simulink model "finalpidsrm"  (R2023a)
settings: Solver=VariableStepAuto  StartTime=0.0  StopTime=10  RelTol=1e-3
undefined symbols (not defined in the file): DiscIntNeverNeededParam
libraries: spsDiodeLib x6, spsIGBTLib x6, spsDCVoltageSourceLib x1, slpidlib x1, spsSwitchedReluctanceMotorLib x1, sps_lib x1
settings Model: Creator=hp  LastModifiedBy=SAGNEEK SENGUPTA
settings SolverCC: ZeroCrossAlgorithm=Adaptive
settings DebuggingCC: IgnoredZcDiagnostic=none

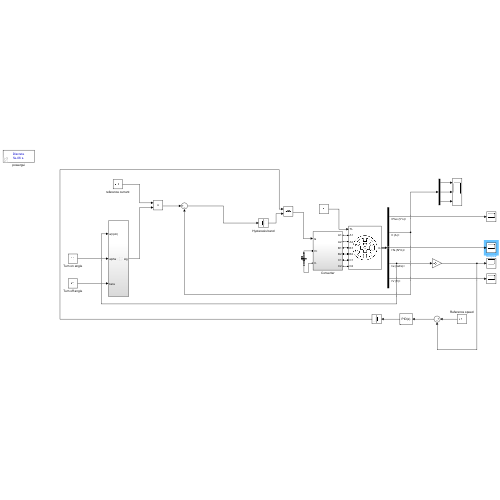
[thumbnail: Simulink's stored preview of the top-level diagram]
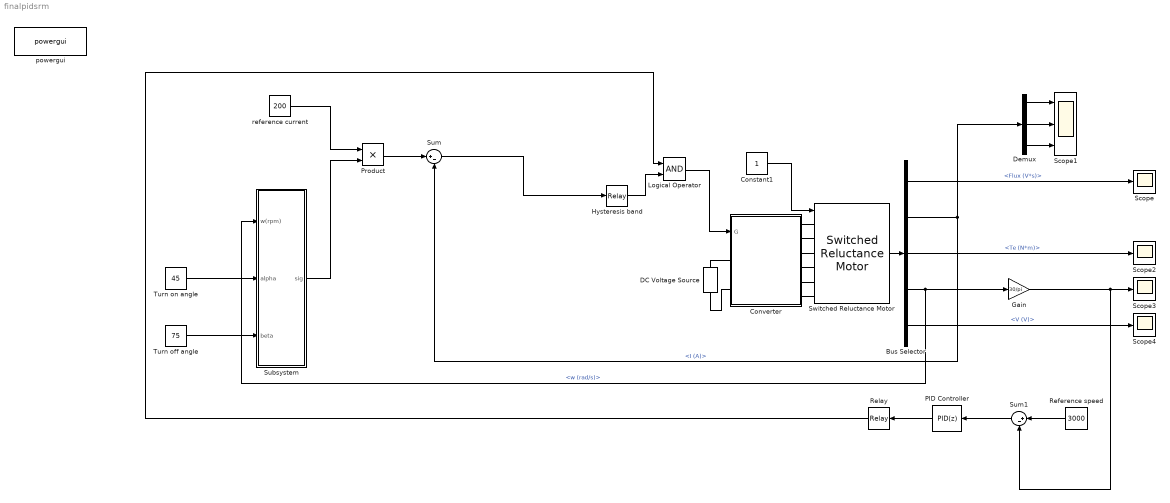
== system finalpidsrm ==
  Bus Selector : BusSelector  OutputSignals=Flux (V*s),I (A),Te (N*m),w (rad/s),V (V)
  Constant1 : Constant
  Converter : Subsystem
  DC Voltage Source : spsDCVoltageSourceLib/DC Voltage Source  Amplitude=240  Measurements=Voltage
  Demux : Demux  Outputs=3
  Gain : Gain  Gain=30/pi
  Hysteresis band : Relay  OnSwitchValue=10  OffSwitchValue=-10  ZeroCross=off
  Logical Operator : Logic  AllPortsSameDT=off  OutDataTypeStr=boolean
  PID Controller : slpidlib/PID Controller  Controller=PID  Form=Parallel  TimeDomain=Discrete-time  UseExternalTs=off  SampleTime=-1  IntegratorMethod=Forward Euler  FilterMethod=Forward Euler  ControllerParametersSource=internal  P=20  I=0.1  UseKiTs=off  D=0.05  N=100  UseFilter=on  TunerSelectOption=Transfer Function Based (PID Tuner App)  InitialConditionSource=internal  InitialConditionForIntegrator=0  InitialConditionForFilter=0  DifferentiatorICPrevScaledInput=0  ExternalReset=none  TrackingMode=off  Kt=1  LimitOutput=off  SatLimitsSource=internal  UpperSaturationLimit=inf  LowerSaturationLimit=-inf  LinearizeAsGain=on  AntiWindupMode=none  Kb=1  LimitIntegrator=off  UpperIntegratorSaturationLimit=inf  LowerIntegratorSaturationLimit=-inf  POutMin=[]  POutMax=[]  IOutMin=[]  IOutMax=[]  DOutMin=[]  DOutMax=[]  NOutMin=[]  NOutMax=[]  SumOutMin=[]  SumOutMax=[]  SaturationOutMin=[]  SaturationOutMax=[]  PParamMin=[]  PParamMax=[]  IParamMin=[]  IParamMax=[]  DParamMin=[]  DParamMax=[]  NParamMin=[]  NParamMax=[]  KbParamMin=[]  KbParamMax=[]  KtParamMin=[]  KtParamMax=[]  KbOutMin=[]  KbOutMax=[]  KtOutMin=[]  KtOutMax=[]  IntegratorOutMin=[]  IntegratorOutMax=[]  FilterOutMin=[]  FilterOutMax=[]  SumI1OutMin=[]  SumI1OutMax=[]  SumI2OutMin=[]  SumI2OutMax=[]  SumI3OutMin=[]  SumI3OutMax=[]  SumI4OutMin=[]  SumI4OutMax=[]  SumDOutMin=[]  SumDOutMax=[]  DifferentiatorOutMin=[]  DifferentiatorOutMax=[]  FilterDiffOutCoefMin=[]  FilterDiffOutCoefMax=[]  ReciprocalOutMin=[]  ReciprocalOutMax=[]  SumDenOutMin=[]  SumDenOutMax=[]  SumNumOutMin=[]  SumNumOutMax=[]  DivideOutMin=[]  DivideOutMax=[]  UdiffTsProdOutMin=[]  UdiffTsProdOutMax=[]  NTsProdOutMin=[]  NTsProdOutMax=[]  UintegralTsProdOutMin=[]  UintegralTsProdOutMax=[]  UngainTsProdOutMin=[]  UngainTsProdOutMax=[]  ClampingZeroOutDataTypeStr=Inherit: Inherit via back propagation  ClampingZeroOutMin=[]  ClampingZeroOutMax=[]  FilterDenConstantOutDataTypeStr=Inherit: Inherit via back propagation  FilterDenConstantOutMin=[]  FilterDenConstantOutMax=[]  PCopyOutDataTypeStr=Inherit: Inherit via back propagation  PCopyOutMin=[]  PCopyOutMax=[]  NCopyOutDataTypeStr=Inherit: Inherit via back propagation  NCopyOutMin=[]  NCopyOutMax=[]  IntegratorContinuousStateAttributes=''  IntegratorStateMustResolveToSignalObject=off  IntegratorRTWStateStorageClass=Auto  FilterContinuousStateAttributes=''  FilterStateMustResolveToSignalObject=off  FilterRTWStateStorageClass=Auto  ParallelPVariant=InternalParameters  IdealPVariant=Disabled  IVariant=InternalParameters  DVariant=InternalParameters  IntegratorVariant=Discrete  SatVariant=Disabled  AWVariant=Passthrough  PCopyVariant=Disabled  TRVariant=Disabled  FdbkBlocksVariant=Forward  IdealPFdbkVariant=Disabled  SatFdbkVariant=Disabled  DerivativeFilterVariant=ForwardEulerFilter  NVariant=InternalParameters  NCopyVariant=Disabled  FilterICVariant=InternalICsFilter  IntegratorICVariant=InternalICs  ExternalResetVariant=Disabled  TRSumVariant=Passthrough  SumFdbkVariant=Disabled  SumVariant=Sum_PID  TsampFilterVariant=InternalTs  TsampNgainVariant=Passthrough  TsampIntegralVariant=Disabled_SignalSpec  ExternalSaturationOutDataTypeStr=Inherit: Same as second input
  Product : Product
  Reference speed : Constant  Value=3000
  Relay : Relay
  Scope{,2..4} (4 alike) : Scope
  Scope1 : Scope  NumInputPorts=3
  Subsystem : Subsystem
  Sum : Sum  Inputs=|+-
  Sum1 : Sum  Inputs=|+-
  Switched Reluctance Motor : spsSwitchedReluctanceMotorLib/Switched Reluctance Motor  MachineType=6/4  StatorResistance=0.08  Inertia=0.0082  Friction=0.05  InitialSpeed=[0 0]  TsPowergui=0  TsBlock=-1  MachineModel=Generic model  Lq=0.67e-3  Ld=23.6e-3  Lsat=0.15e-3  MaximumCurrent=90  MaximumFluxLinkage=0.486  Source=MAT-file  MagnetisationCharacteristic='srm64_60kw.mat'  RotorAngleVector=[0 10 20 30 40 45]  StatorCurrentVector=[0:25:450]  PlotCurves=off
      settings: LibrarySourceBlock=|
      | sps_lib/Electrical Machines/Switched Reluctance
      | Motor
  Turn off angle : Constant  Value=75
  Turn on angle : Constant  Value=45
  powergui : sps_lib/powergui  Priority=1  SimulationMode=Discrete  SampleTime=5e-06  frequency=60  Iterations=50  frequencyindice=0  Pbase=100e6  ErrMax=1e-4  UnitsV=kV  UnitsW=MW  buscounter=0  FunctionMessages=off  echomessages=off  EnableUseOfTLC=off  CurrentSourceSwitches=off  DisableSnubberDevices=off  DisableRonSwitches=off  DisableVfSwitches=off  DisplayEquations=off  AutomaticDiscreteSolvers=off  SolverType=Tustin/Backward Euler (TBE)  Interpol=off  ExternalGateDelay=off  methode=off  Ts=100  x0status=blocks  SPID=on  SwTol=0  HookPort=off  NonlinearTolerance=1e-4  nMaxIteration=100  ContinueOnMaxIteration=off  RestoreLinks=warning  ResistiveCurrentMeasurement=off  Frange=[0:2:500]  Ylog=off  Xlog=on  ShowGrid=off  save=off  variable=ZData  structure=0  ZoomFFT=off  StartTime=0.0  cycles=1  DisplayStyle=1  fundamental=60  FreqAxis=off  MaxFrequency=1000  frequencyindicesteady=1  RmsSteady=1  display=off
  reference current : Constant  Value=200
  wires:
  Bus Selector/4 -> Subsystem/1(w(rpm)), Gain/1  "<w (rad/s)>"
  Gain/1 -> Scope3/1, Sum1/2
  Switched Reluctance Motor/1 -> Bus Selector/1
  Constant1/1 -> Switched Reluctance Motor/1
  Bus Selector/1 -> Scope/1  "<Flux (V*s)>"
  Bus Selector/2 -> Sum/2, Demux/1  "<I (A)>"
  Turn on angle/1 -> Subsystem/2(alpha)
  Turn off angle/1 -> Subsystem/3(beta)
  Subsystem/1(sig) -> Product/2
  reference current/1 -> Product/1
  Sum/1 -> Hysteresis band/1
  Product/1 -> Sum/1
  Reference speed/1 -> Sum1/1
  Sum1/1 -> PID Controller/1
  PID Controller/1 -> Relay/1
  Hysteresis band/1 -> Logical Operator/2
  Relay/1 -> Logical Operator/1
  Logical Operator/1 -> Converter/1(G)
  Demux/1 -> Scope1/1
  Demux/2 -> Scope1/2
  Demux/3 -> Scope1/3
  Bus Selector/3 -> Scope2/1  "<Te (N*m)>"
  Bus Selector/5 -> Scope4/1  "<V (V)>"
  connections:
  Converter/LConn1 -- DC Voltage Source/RConn1
  DC Voltage Source/LConn1 -- Converter/LConn2
  Converter/RConn5 -- Switched Reluctance Motor/LConn5
  Converter/RConn3 -- Switched Reluctance Motor/LConn3
  Converter/RConn2 -- Switched Reluctance Motor/LConn2
  Converter/RConn1 -- Switched Reluctance Motor/LConn1
  Converter/RConn6 -- Switched Reluctance Motor/LConn6
  Converter/RConn4 -- Switched Reluctance Motor/LConn4

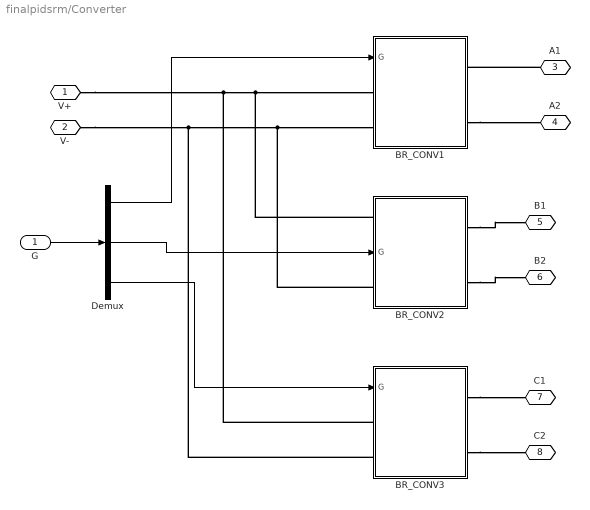
== system finalpidsrm/Converter ==
  G : Inport
  BR_CONV1 : Subsystem
  BR_CONV2 : Subsystem
      settings: PortSchema="{\"entries\":[{\"content\":{\"sides\":[{\"content\":{\"connectorIds\":[\"LConn1\",\"In1\",\"LConn2\"]},\"type\":\"ConnectorPlacement.EquallySpacedRectSide\",\"uuid\":\"faabb453-bb22-4931-9e9b-92bf35074774\"},{\"content\":{\"connectorIds\":[\"RConn1\",\"RConn2\"],\"side\":\"RIGHT\"},\"type\":\"ConnectorPlacement.EquallySpacedRectSide\",\"uuid\":\"a34aaca4-6214-4530-a60a-d4498c83c57f\"},{\"content\":{\"side\":\"TOP\"},\"type\":\"ConnectorPlacement.EquallySpacedRectSide\",\"uuid\":\"9aa06430-66ef-4358-b98b-d7ce8e74a211\"}]},\"type\":\"ConnectorPlacement.EquallySpacedConnector\",\"uuid\":\"ce43af93-db24-45ea-bfee-aa3632ef56a0\"}],\"packageUris\":[\"http://schema.mathworks.com/mf0/Connector/R2020b\"],\"version\":\"1.0\"}"
  BR_CONV3 : Subsystem
  Demux : Demux  Outputs=3
  V+ : PMIOPort  Side=Left
  V- : PMIOPort  Port=2  Side=Left
  A1 : PMIOPort  Port=3  Side=Right
  A2 : PMIOPort  Port=4  Side=Right
  B1 : PMIOPort  Port=5  Side=Right
  B2 : PMIOPort  Port=6  Side=Right
  C1 : PMIOPort  Port=7  Side=Right
  C2 : PMIOPort  Port=8  Side=Right
  wires:
  G/1 -> Demux/1
  Demux/1 -> BR_CONV1/1(G)
  Demux/2 -> BR_CONV2/1(G)
  Demux/3 -> BR_CONV3/1(G)
  connections:
  V+/RConn1 -- BR_CONV3/LConn1 -- BR_CONV2/LConn1 -- BR_CONV1/LConn1
  V-/RConn1 -- BR_CONV3/LConn2 -- BR_CONV2/LConn2 -- BR_CONV1/LConn2
  A1/RConn1 -- BR_CONV1/RConn1
  BR_CONV1/RConn2 -- A2/RConn1
  BR_CONV2/RConn1 -- B1/RConn1
  BR_CONV2/RConn2 -- B2/RConn1
  BR_CONV3/RConn1 -- C1/RConn1
  BR_CONV3/RConn2 -- C2/RConn1

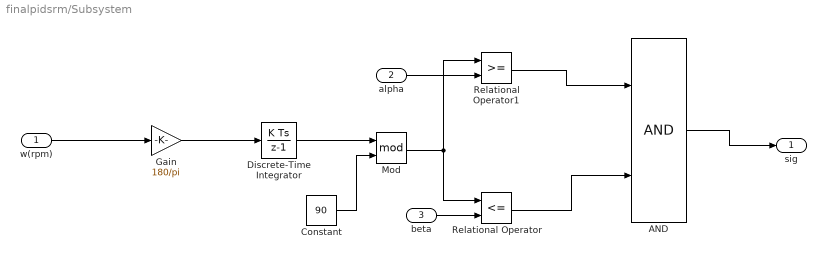
== system finalpidsrm/Subsystem ==
  w(rpm) : Inport
  alpha : Inport  Port=2
  beta : Inport  Port=3
  AND : Logic  AllPortsSameDT=off  OutDataTypeStr=boolean
  Constant : Constant  Value=90
  Discrete-Time Integrator : DiscreteIntegrator  InitialCondition=[0 -30 -60]  SampleTime=5e-06  ICPrevOutput=DiscIntNeverNeededParam  ICPrevScaledInput=DiscIntNeverNeededParam
  Gain : Gain  Gain=180/pi
  Mod : Math  Operator=mod
  Relational Operator : RelationalOperator  Operator=<=  OutDataTypeStr=boolean  RndMeth=Simplest  InputSameDT=off
  Relational Operator1 : RelationalOperator  OutDataTypeStr=boolean  RndMeth=Simplest  InputSameDT=off
  sig : Outport
  wires:
  Gain/1 -> Discrete-Time Integrator/1
  beta/1 -> Relational Operator/2
  Constant/1 -> Mod/2
  Discrete-Time Integrator/1 -> Mod/1
  Mod/1 -> Relational Operator1/1, Relational Operator/1
  AND/1 -> sig/1
  w(rpm)/1 -> Gain/1
  alpha/1 -> Relational Operator1/2
  Relational Operator1/1 -> AND/1
  Relational Operator/1 -> AND/2

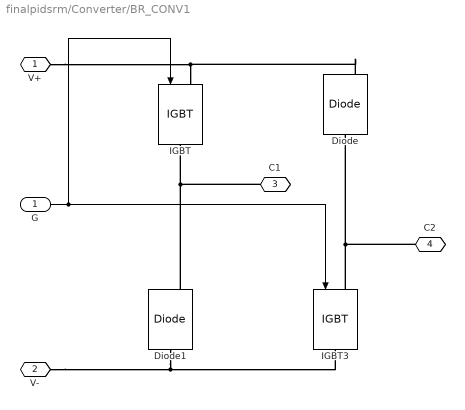
== system finalpidsrm/Converter/BR_CONV1 ==
  G : Inport
  Diode : spsDiodeLib/Diode  Ron=0.001  Lon=0  Vf=0.8  IC=0  UseSnubber=0  Rs=1000  Cs=inf  Measurements=on
  Diode1 : spsDiodeLib/Diode  Ron=0.001  Lon=0  Vf=0.8  IC=0  UseSnubber=0  Rs=1000  Cs=inf  Measurements=on
  IGBT : spsIGBTLib/IGBT  Ron=1e-3  Lon=0  Vf=1  Tf=1e-6  Tt=2e-6  IC=0  Rs=200  Cs=0.1e-6  Measurements=off
  IGBT3 : spsIGBTLib/IGBT  Ron=1e-3  Lon=0  Vf=1  Tf=1e-6  Tt=2e-6  IC=0  Rs=200  Cs=0.1e-6  Measurements=off
  V+ : PMIOPort  Side=Left
  V- : PMIOPort  Port=2  Side=Left
  C1 : PMIOPort  Port=3  Side=Right
  C2 : PMIOPort  Port=4  Side=Right
  wires:
  G/1 -> IGBT3/1, IGBT/1
  connections:
  V+/RConn1 -- Diode/RConn1 -- IGBT/LConn1
  C2/RConn1 -- Diode/LConn1 -- IGBT3/LConn1
  C1/RConn1 -- IGBT/RConn1 -- Diode1/RConn1
  V-/RConn1 -- Diode1/LConn1 -- IGBT3/RConn1

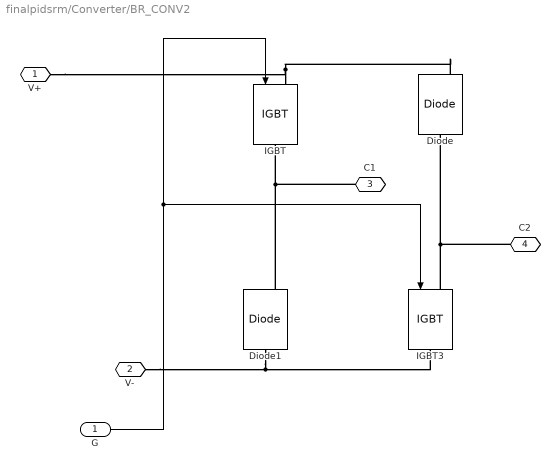
== system finalpidsrm/Converter/BR_CONV2 ==
  G : Inport
  Diode : spsDiodeLib/Diode  Ron=0.001  Lon=0  Vf=0.8  IC=0  UseSnubber=0  Rs=1000  Cs=inf  Measurements=on
  Diode1 : spsDiodeLib/Diode  Ron=0.001  Lon=0  Vf=0.8  IC=0  UseSnubber=0  Rs=1000  Cs=inf  Measurements=on
  IGBT : spsIGBTLib/IGBT  Ron=1e-3  Lon=0  Vf=1  Tf=1e-6  Tt=2e-6  IC=0  Rs=200  Cs=0.1e-6  Measurements=off
  IGBT3 : spsIGBTLib/IGBT  Ron=1e-3  Lon=0  Vf=1  Tf=1e-6  Tt=2e-6  IC=0  Rs=200  Cs=0.1e-6  Measurements=off
  V+ : PMIOPort  Side=Left
  V- : PMIOPort  Port=2  Side=Left
  C1 : PMIOPort  Port=3  Side=Right
  C2 : PMIOPort  Port=4  Side=Right
  wires:
  G/1 -> IGBT/1, IGBT3/1
  connections:
  C1/RConn1 -- IGBT/RConn1 -- Diode1/RConn1
  C2/RConn1 -- Diode/LConn1 -- IGBT3/LConn1
  IGBT/LConn1 -- Diode/RConn1 -- V+/RConn1
  V-/RConn1 -- Diode1/LConn1 -- IGBT3/RConn1

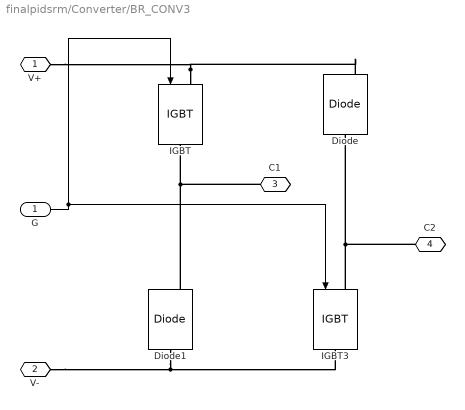
== system finalpidsrm/Converter/BR_CONV3 ==
  G : Inport
  Diode : spsDiodeLib/Diode  Ron=0.001  Lon=0  Vf=0.8  IC=0  UseSnubber=0  Rs=1000  Cs=inf  Measurements=on
  Diode1 : spsDiodeLib/Diode  Ron=0.001  Lon=0  Vf=0.8  IC=0  UseSnubber=0  Rs=1000  Cs=inf  Measurements=on
  IGBT : spsIGBTLib/IGBT  Ron=1e-3  Lon=0  Vf=1  Tf=1e-6  Tt=2e-6  IC=0  Rs=200  Cs=0.1e-6  Measurements=off
  IGBT3 : spsIGBTLib/IGBT  Ron=1e-3  Lon=0  Vf=1  Tf=1e-6  Tt=2e-6  IC=0  Rs=200  Cs=0.1e-6  Measurements=off
  V+ : PMIOPort  Side=Left
  V- : PMIOPort  Port=2  Side=Left
  C1 : PMIOPort  Port=3  Side=Right
  C2 : PMIOPort  Port=4  Side=Right
  wires:
  G/1 -> IGBT3/1, IGBT/1
  connections:
  C1/RConn1 -- IGBT/RConn1 -- Diode1/RConn1
  C2/RConn1 -- Diode/LConn1 -- IGBT3/LConn1
  IGBT/LConn1 -- V+/RConn1 -- Diode/RConn1
  V-/RConn1 -- IGBT3/RConn1 -- Diode1/LConn1
